simulink model "car_model_FIXED"  (R2022b)
settings: Solver=VariableStepAuto  StartTime=0.0  StopTime=60  RelTol=1e-3
values from neighbouring files (symbols this model uses):
  ABS_MAX_TORQUE = [25 25 25 25]    [workspace.mat]
  ABS_MAX_TRQ_CMD = 50    [workspace.mat]
  ABS_MIN_TORQUE = [0.01 0.01 0.01 0.01]    [workspace.mat]
  acc_IC = 0    [workspace.mat]
  ACCELERATION_MAX = 30    [workspace.mat]
  ActSuspDutyCycle = 1    [workspace.mat]
  Aeq_left = [0.305756190204 0.308857786592 0.311945941182 0.315020811431 0.318082554689 0.321131328186 0.324167289011 0.327190594103 0.330201400225 0.333199863958 0.336186141681 0.339160389558 ... (261 elements, 1x261)]    [workspace.mat]
  Aeq_right = [-0.961664782545 -0.959835898365 -0.957982924115 -0.956106413788 -0.954206913862 -0.952284963337 -0.950341093764 -0.948375829284 -0.946389686656 -0.944383175301 -0.942356797333 -0.940311047601 ... (261 elements, 1x261)]    [workspace.mat]
  alpha_error = 0.1    [workspace.mat]
  ang_acc_hystersesis = 0.1    [workspace.mat]
  ang_IC = 0    [workspace.mat]
  ang_vel_IC = 0    [workspace.mat]
  area_air = 0.15    [workspace.mat]
  axb = -5    [workspace.mat]
  battery_current_IC = 0    [workspace.mat]
  BATTERY_CURRENT_MAX = 140    [workspace.mat]
  BATTERY_CURRENT_MIN = 0    [workspace.mat]
  battery_FT_IC = 300    [workspace.mat]
  battery_T_IC = 300    [workspace.mat]
  BATTERY_TEMPERATURE_MAX = 60    [workspace.mat]
  BATTERY_TEMPERATURE_MIN = 0    [workspace.mat]
  battery_voltage_IC = 332    [workspace.mat]
  BATTERY_VOLTAGE_MAX = 340    [workspace.mat]
  BATTERY_VOLTAGE_MIN = 60    [workspace.mat]
  br = 0.01    [workspace.mat]
  brake_bias = [0.35 0.35 0.15 0.15]    [workspace.mat]
  Brake_Pressure_IC = 1    [workspace.mat]
  ccl_IC = 0    [workspace.mat]
  CENTER_STEER_ANGLE_MAX = 130    [workspace.mat]
  covarience_matrix_IC = [0.001 0 0 0 0 0 0 0 0 0 0 0 ... (784 elements, 28x28)]    [workspace.mat]
  CURRENT_BUFFER = 25    [workspace.mat]
  cy_sweep = [13568.4166816 14020.2069783 14456.754831 14879.7402576 15289.7264712 15687.2766846 16072.954111 16447.3219632 16810.9434544 17164.3817975 17508.2002054 17842.9618912 ... (101 elements, 1x101)]    [workspace.mat]
  dB = 0.001    [workspace.mat]
  dcl_IC = 140    [workspace.mat]
  DCL_MAX = 130    [workspace.mat]
  DCL_MIN = 0    [workspace.mat]
  deadband_angle = 12    [workspace.mat]
  dIndex = 50    [workspace.mat]
  driver_t = 0.015    [workspace.mat]
  dt_OFF = 4.5    [workspace.mat]
  dt_ON = 7.5    [workspace.mat]
  dTx = 0.01    [workspace.mat]
  dx = 0.1    [workspace.mat]
  dZ = 0.295    [workspace.mat]
  efficiency_grid = [0.759500051293 0.787587791453 0.809832189108 0.826747821898 0.837164543102 0.842744381136 0.842258400104 0.838611650621 0.82826195101 0.814029316176 0.795690627225 0.7759791486 ... (2782 elements, 26x107)]    [workspace.mat]
  F0z = [0 0]    [workspace.mat]
  forward_look_straight = 5    [workspace.mat]
  forward_look_turn = 15    [workspace.mat]
  Fz_IC = 539.55    [workspace.mat]
  Fz_sweep = [200 210 220 230 240 250 260 270 280 290 300 310 ... (101 elements, 1x101)]    [workspace.mat]
  g = 9.81    [workspace.mat]
  GAIN_ABS = 100    [workspace.mat]
  gearbox_efficiency = [0.8 0.8 0.8 0.8]    [workspace.mat]
  gps_counter_IC = 0    [workspace.mat]
  gps_hz = 0.01    [workspace.mat]
  gr = [8.74786324786 8.74786324786 8.74786324786 8.74786324786]    [workspace.mat]
  I = 0    [workspace.mat]
  I_Driver = 1    [workspace.mat]
  indicies = [3 3.5 4 0.5 1 1.5 2 2.5 3 3.5 4 0.5 ... (27 elements, 1x27)]    [workspace.mat]
  IYY = 0.3    [workspace.mat]
  kx_sweep = [8779.958 9178.302 9576.646 9974.99 10373.334 10771.678 11170.022 11568.366 11966.71 12365.054 12763.398 13161.742 ... (101 elements, 1x101)]    [workspace.mat]
  l = [0.772 0.772]    [workspace.mat]
  lambda_star = 0.15    [workspace.mat]
  low_V_SA = 0.001    [workspace.mat]
  lr = 35    [workspace.mat]
  m_all = 220    [workspace.mat]
  m_body = 180    [workspace.mat]
  m_unsprung = [6 6 14 14]    [workspace.mat]
  MAG_MAX = 200    [workspace.mat]
  Max_Brake_Pressure = 100000000    [workspace.mat]
  Max_Driver_Input = 1    [workspace.mat]
  MAX_DTHETA_DRIVER = 360    [workspace.mat]
  MAX_I_Driver = 1    [workspace.mat]
  MAX_STEERING_ADJUST = 15    [workspace.mat]
  max_yaw = [0.705271610162 0.928228152446 1.12280857731 1.14131008363 1.08727026041 1.01377803859 0.938114723816 0.8718206875 0.815009168116 0.767481919497 0.727119764215 0.694403589394 ... (15 elements, 1x15)]    [workspace.mat]
  Min_Brake_Pressure = 1    [workspace.mat]
  Min_Driver_Input = 0    [workspace.mat]
  min_velocity_regen = 1.4    [workspace.mat]
  motor_current_IC = 0    [workspace.mat]
  MOTOR_CURRENT_MAX = 70    [workspace.mat]
  MOTOR_CURRENT_MIN = 0    [workspace.mat]
  MOTOR_ENABLE = [0 0 1 1]    [workspace.mat]
  motor_FT_IC = 300    [workspace.mat]
  motor_T_IC = 300    [workspace.mat]
  MOTOR_TEMPERATURE_MAX = 100    [workspace.mat]
  MOTOR_TEMPERATURE_MIN = 0    [workspace.mat]
  motor_voltage_IC = 332    [workspace.mat]
  MOTOR_VOLTAGE_MAX = 340    [workspace.mat]
  MOTOR_VOLTAGE_MIN = 90    [workspace.mat]
  motorControllerCurve = [25  260; 50  130; 75  0]    [workspace.mat]
  motorTempCurve = [140 138.6 134.4 127.4 117.6 105 89.6 71.4 50.4 26.6 0]    [workspace.mat]
  motorTempX = [75 77 79 81 83 85 87 89 91 93 95]    [workspace.mat]
  mu_star = 0.5    [workspace.mat]
  mx_sweep = [3.38348 3.3655067 3.3477908 3.3303323 3.3131312 3.2961875 3.2795012 3.2630723 3.2469008 3.2309867 3.21533 3.1999307 ... (101 elements, 1x101)]    [workspace.mat]
  my_sweep = [3.036232 3.015241699 2.994987032 2.975452753 2.956623616 2.938484375 2.921019784 2.904214597 2.888053568 2.872521451 2.857603 2.843282969 ... (101 elements, 1x101)]    [workspace.mat]
  noise_state = [1e-06 1e-06 1e-06 1e-06 0.005 0.005 0.005 1e-06 1e-06 1e-06 1e-06 1e-06 ... (28 elements, 28x1)]    [workspace.mat]
  omega_IC = 0    [workspace.mat]
  OMEGA_MAX = 150    [workspace.mat]
  OMEGA_MIN = 0    [workspace.mat]
  ORIENTATION_MAX = 360    [workspace.mat]
  P = 2    [workspace.mat]
  P_Driver = 0.7    [workspace.mat]
  P_High_Speed = 0.1    [workspace.mat]
  P_Steering_Adjust = 2    [workspace.mat]
  P_Straight_Adjust = 5    [workspace.mat]
  pos_IC = 0    [workspace.mat]
  POS_MAX = 300    [workspace.mat]
  q_thresh = 0.3    [workspace.mat]
  RE = 0.223    [workspace.mat]
  rho = 1.225    [workspace.mat]
  s = [0.649 0.621]    [workspace.mat]
  selected_maxvm = [49.86390724 16.21289794 8.219813569 8.05215527 7.103352929 8.35634983 13.87515039 8.72402841 22.75224945 36.67909339 19.32001297 25.09036962 ... (63 elements, 21x3)]    [workspace.mat]
  selected_sweep = [3 3 3 3 3 3 3 3 3 3 3 3 ... (1288 elements, 644x2)]    [workspace.mat]
  selected_track = [inf inf inf inf inf inf inf inf inf inf inf inf ... (37971 elements, 4219x9)]    [workspace.mat]
  shock_length_IC = 0.1    [workspace.mat]
  SHOCK_LENGTH_MAX = 0.25    [workspace.mat]
  SHOCK_LENGTH_MIN = 0    [workspace.mat]
  state_IC = [1 0 0 0 0 0 0 0 0 0 0 0 ... (28 elements, 28x1)]    [workspace.mat]
  steering_sweep = [0 5 10 15 20 25 30 35 40 45 50 55 ... (27 elements, 1x27)]    [workspace.mat]
  steering_Up_Grid = [0.551231966244 8.36038106007 16.1333806643 23.9559539118 31.8240691982 39.7561724339 47.7157531433 55.7845698794 64.1341708168 73.0798046026 82.7903081349 93.1297322155 ... (615 elements, 41x15)]    [workspace.mat]
  ... (+25 more)
undefined symbols (not defined in the file or in its folder): ax, ay, az, covA, covG, covM, covP, covV, DiscIntNeverNeededParam, fusion_t, fusion_t_sim, gps_ratio, IMU_accel, IMU_gyro, imu_hz, IMU_mag, location_lla_IC, p, phi, psi, q, r, sus, theta, trn, veh, VEH, whl, X, Xdot, Y, Ydot, Z, Zdot
libraries: fl_lib x82, nesl_utility x32, vehdynlibtire x10, vehdynlibsuspension x8, simulink x5, autolibutils x5, sharedtransform x5, sdl_lib x4, EngineCoolingComponents_lib x4, slpidlib x3, SimscapeFluids_lib x3, shared6dof x2
(part 4 of 14)

== system car_model_FIXED/Vehicle Model/Suspension ==
  Steering : Inport
  Wheel : Inport  Port=2
  Vehicle : Inport  Port=3
  Double Wishbone Suspension : Subsystem  VariantControl=1
      mask Display: image('suspdw.png');
  Independent Mapped Front Suspension Mapped Solid Axle Rear Suspension : Subsystem  VariantControl=2
      mask Display: image([imread('suspindmap.png');imread('suspsamap.png')]);
  Kinematics and Compliance Independent Suspension : Subsystem  VariantControl=6
      mask Display: image('suspkandc.png');
  MacPherson Front Suspension Solid Axle Rear Suspension : Subsystem  VariantControl=3
      mask Display: image([imread('suspmacp.png');imread('suspsacoil.png')]);
  MacPherson Suspension : Subsystem  VariantControl=4
      mask Display: image('suspmacp.png');
  Mapped Suspension : Subsystem  VariantControl=5
      mask Display: image('suspindmap.png');
  Suspension : Outport  VectorParamsAs1DForOutWhenUnconnected=off
  Suspension1 : Outport  Port=2  VectorParamsAs1DForOutWhenUnconnected=off
  Veh : Outport  Port=3  VectorParamsAs1DForOutWhenUnconnected=off

== system car_model_FIXED/Vehicle Model/Vehicle ==
  Suspension : Inport
  6DOF : Subsystem  VariantControl=1
  Constant : Constant  Value=[0 0 0]
  VehFdbk : Outport  VectorParamsAs1DForOutWhenUnconnected=off
  wires:
  6DOF/1(VehFdbk) -> VehFdbk/1  "VehFdbk"
  Constant/1 -> 6DOF/2(Wind)
  Suspension/1 -> 6DOF/1(Suspension)

== system car_model_FIXED/Vehicle Model/Wheels and Tires ==
  Brake Press : Inport  Unit=Pa
  PwrTrn : Inport  Port=2
  Sus : Inport  Port=3
  Veh : Inport  Port=4
  Bus Selector : BusSelector  OutputSignals=axle_torque
  Bus Selector1 : BusSelector  OutputSignals=Whl.Ang,Whl.F,Whl.AngVel,Whl.xdot,Whl.ydot
  Bus Selector2 : BusSelector  OutputSignals=BdyFrm.Cg.Vel.xdot,BdyFrm.Cg.Vel.ydot  OutputAsBus=on
  Constant1 : Constant  Value=[1 1 1 1].*0.00182
  Constant3 : Constant  Value=[1 1 1 1]
  Cont LPF : autolibutils/Cont LPF  wc=100*2*pi  AbsoluteTolerance=auto  aMode=2
  Cont LPF1 : autolibutils/Cont LPF  wc=100*2*pi  AbsoluteTolerance=auto  aMode=2
  Matrix Concatenate : Concatenate  NumInputs=3  Mode=Multidimensional array
  Reshape{1..4} (4 alike) : Reshape
  Saturation : Saturate  UpperLimit=inf  LowerLimit=-10*9.81*2000  ZeroCross=off
  Selector : Selector  NumberOfDimensions=2  InputPortWidth=3  IndexOptions=Index vector (dialog),Select all  Indices=[3],1  OutputSizes=1,1
  Selector1 : Selector  NumberOfDimensions=2  InputPortWidth=1  IndexOptions=Index vector (dialog),Select all  Indices=[3],1  OutputSizes=1,1
  Selector2 : Selector  NumberOfDimensions=2  InputPortWidth=3  IndexOptions=Index vector (dialog),Select all  Indices=3,1  OutputSizes=1,1
  Selector3 : Selector  NumberOfDimensions=2  InputPortWidth=3  IndexOptions=Index vector (dialog),Select all  Indices=1,1  OutputSizes=1,1
  Sqrt : Sqrt
  Square : Math  Operator=square
  Sum : Sum  Inputs=+
  Terminator{,1..2,4..5} (5 alike) : Terminator
  VDBS : Subsystem  VariantControl=0
  Vehicle : Outport  VectorParamsAs1DForOutWhenUnconnected=off
  Suspension : Outport  Port=2  VectorParamsAs1DForOutWhenUnconnected=off
  Wheels : Outport  Port=3  VectorParamsAs1DForOutWhenUnconnected=off
  Power Train : Outport  Port=4  VectorParamsAs1DForOutWhenUnconnected=off
  Wheels2Susp : Outport  Port=5  VectorParamsAs1DForOutWhenUnconnected=off
  Vg : Outport  Port=6  VectorParamsAs1DForOutWhenUnconnected=off
  wires:
  Bus Selector1/2 -> Selector/1  "<F>"
  VDBS/3(FrntAxlF) -> Terminator/1
  VDBS/4(RearAxlF) -> Terminator1/1
  VDBS/6(Mz) -> Terminator4/1
  Selector1/1 -> Reshape1/1
  Matrix Concatenate/1 -> VDBS/7(VehVel)
  PwrTrn/1 -> Power Train/1, Bus Selector/1
  Reshape4/1 -> VDBS/1(WhlAng)  "WhlAng"
  Reshape3/1 -> VDBS/2(WhlCmb)  "WhlCmb"
  Selector/1 -> Reshape2/1
  Saturation/1 -> VDBS/5(Fz)
  Constant1/1 -> VDBS/8(Ground Level)
  VDBS/8(SuspWhlVz) -> Matrix Concatenate/3  "zdot"
  Bus Selector1/1 -> Cont LPF1/1  "<Ang>"
  Selector3/1 -> Reshape3/1  "Camber Angles"
  Sus/1 -> Suspension/1, Bus Selector1/1
  Bus Selector1/4 -> Matrix Concatenate/1  "<xdot>"
  Bus Selector1/5 -> Matrix Concatenate/2  "<ydot>"
  VDBS/7(SuspWhlPz) -> Terminator5/1  "z"
  Reshape2/1 -> Cont LPF/1
  Bus Selector1/3 -> Selector1/1  "<AngVel>"
  Reshape1/1 -> VDBS/6(r)
  Brake Press/1 -> VDBS/4(BrkPed)
  Constant3/1 -> VDBS/9(Friction)
  Cont LPF/1 -> Saturation/1
  Cont LPF1/1 -> Selector3/1, Selector2/1
  Selector2/1 -> Reshape4/1  "Wheel Angles"
  Veh/1 -> Vehicle/1, Bus Selector2/1, VDBS/10(Veh)  "Veh"
  VDBS/2(Wheels2Susp) -> Wheels2Susp/1  "Wheels"
  VDBS/1(Wheels) -> Wheels/1
  Bus Selector/1 -> VDBS/3(AxleTrq)  "<axle_torque>"
  VDBS/5(Omega) -> Terminator2/1
  Bus Selector2/1 -> Square/1
  Square/1 -> Sum/1
  Sum/1 -> Sqrt/1
  Sqrt/1 -> Vg/1

== system car_model_FIXED/Control Systems/TVS/Optimization ==
  note: reduce this limit?
  driver_input : Inport  OutDataTypeStr=double
  obj_gain : Inport  Port=2
  b : Inport  Port=3  OutDataTypeStr=double
  ub : Inport  Port=4  OutDataTypeStr=double
  lb : Inport  Port=5  OutDataTypeStr=double
  Aeq : Inport  Port=6  OutDataTypeStr=double
  beq : Inport  Port=7  OutDataTypeStr=double
  A Dot : DotProduct  OutDataTypeStr=double
  Aeq Dot : DotProduct  OutDataTypeStr=double
  C Caller : CCaller  FunctionName=bigM_func  PortSpecificationStruct="%)30     .    N\"X   8    (     @         %    \"    !P    !     0         %  0 \"0    $    _    07)G3F%M90  4&]R=$YA;64 4V-O<&4     26YD97@     5'EP90      4VEZ90      27-';&]B86P   X    P    !@    @    $          4    (     0    ,    !         !   P!O=70 #@   #     &    \"     0         !0    @    !     P    $         $  # &]U=  .    .     8    (    !          %    \"     $    &     0         0  ...(+15750 chars)"
  Constant : Constant  Value=TVS_ENABLE
  Constant1 : Constant  Value=[1 1 1 1]
  Demux{,1..4} (5 alike) : Demux
  Switch : Switch  Criteria=u2 > Threshold  SaturateOnIntegerOverflow=off  InputSameDT=off
  Tx_RAW_demux : Mux
  Tx_choose : Switch  Criteria=u2 > Threshold  Threshold=2  OutDataTypeStr=double  SaturateOnIntegerOverflow=off  InputSameDT=off
  Tx_deadband : DeadZone  LowerValue=-10*dTx  UpperValue=10*dTx  SaturateOnIntegerOverflow=off
  Tx_equal_gain : Gain  Gain=ABS_MAX_TORQUE.*MOTOR_ENABLE  OutDataTypeStr=double
  Tx_equal_offset : Bias  Bias=ABS_MAX_TORQUE  SaturateOnIntegerOverflow=off
  Tx_initial : Constant  Value=Tx_I  OutDataTypeStr=double
  Tx_rate_limit : RateLimiter  RisingSlewLimit=Torque_Up_Rate_Limit  FallingSlewLimit=-Torque_Down_Rate_Limit  SampleTimeMode=inherited
  Tx_reverse_offset : Bias  Bias=-ABS_MAX_TORQUE  SaturateOnIntegerOverflow=off
  b Add : Sum  OutDataTypeStr=double
  beq Add : Sum  OutDataTypeStr=double
  lb_offset : Bias  Bias=ABS_MAX_TORQUE  SaturateOnIntegerOverflow=off
  optimization_offset_A : Constant  Value=ABS_MAX_TORQUE  OutDataTypeStr=double
  optimization_offset_Aeq : Constant  Value=ABS_MAX_TORQUE  OutDataTypeStr=double
  ub_offset : Bias  Bias=ABS_MAX_TORQUE  SaturateOnIntegerOverflow=off
  yaw_error_limit : Constant  Value=yaw_error_limit  OutDataTypeStr=double
  Tx : Outport
  exitflag : Outport  Port=2
  wires:
  C Caller/1 -> Tx_choose/2, exitflag/1  "exitflag"
  lb/1 -> lb_offset/1  "lb"
  ub/1 -> ub_offset/1  "ub"
  C Caller/2 -> Tx_RAW_demux/1  "TFL"
  C Caller/5 -> Tx_RAW_demux/4  "TRR"
  C Caller/4 -> Tx_RAW_demux/3  "TRL"
  C Caller/3 -> Tx_RAW_demux/2  "TFR"
  Demux/1 -> C Caller/1  "obj_FL"
  Demux/2 -> C Caller/2  "obj_FR"
  Demux/3 -> C Caller/3  "obj_RL"
  Demux/4 -> C Caller/4  "obj_RR"
  Tx_initial/1 -> C Caller/23, C Caller/24, C Caller/26, C Caller/25  "Tx_initial"
  Demux1/1 -> C Caller/19  "ub_FL"
  Demux1/2 -> C Caller/20  "ub_FR"
  Demux1/3 -> C Caller/21  "ub_RL"
  Demux1/4 -> C Caller/22  "ub_RR"
  Demux2/1 -> C Caller/15  "lb_FL"
  Demux2/2 -> C Caller/16  "lb_FR"
  Demux2/3 -> C Caller/17  "lb_RL"
  Demux2/4 -> C Caller/18  "lb_RR"
  Demux3/3 -> C Caller/13  "Aeq_RL"
  Demux3/2 -> C Caller/12  "Aeq_FR"
  Demux3/1 -> C Caller/11  "Aeq_FL"
  Demux3/4 -> C Caller/14  "Aeq_RR"
  Demux4/1 -> C Caller/6  "A_FL"
  Demux4/2 -> C Caller/7  "A_FR"
  Demux4/3 -> C Caller/8  "A_RL"
  Demux4/4 -> C Caller/9  "A_RR"
  ub_offset/1 -> Demux1/1  "ub_b"
  optimization_offset_Aeq/1 -> Aeq Dot/1  "offset"
  optimization_offset_A/1 -> A Dot/1  "offset"
  beq/1 -> beq Add/1  "beq"
  Aeq Dot/1 -> beq Add/2  "Aeq_b"
  b/1 -> b Add/1  "b"
  A Dot/1 -> b Add/2
  yaw_error_limit/1 -> C Caller/27  "yaw_error_limit"
  Tx_RAW_demux/1 -> Tx_choose/1  "Tx_RAW_TV"
  Constant1/1 -> Demux4/1, A Dot/2  "A"
  b Add/1 -> C Caller/5  "b_b"
  obj_gain/1 -> Demux/1  "obj_gain"
  lb_offset/1 -> Demux2/1  "lb_b"
  Aeq/1 -> Demux3/1, Aeq Dot/2  "Aeq"
  beq Add/1 -> C Caller/10  "beq_b"
  Tx_rate_limit/1 -> Tx/1  "Tx"
  Tx_reverse_offset/1 -> Tx_deadband/1
  driver_input/1 -> Tx_equal_gain/1
  Tx_deadband/1 -> Tx_rate_limit/1
  Tx_choose/1 -> Switch/1
  Tx_equal_gain/1 -> Tx_equal_offset/1  "Tx_equal"
  Tx_equal_offset/1 -> Switch/3, Tx_choose/3
  Switch/1 -> Tx_reverse_offset/1
  Constant/1 -> Switch/2

== system car_model_FIXED/Control Systems/TVS/Power Controller ==
  note: Tune the distance before PL is enabled
  note: Create a better map wherein you have T,V,I,w
  note: Tune the endpoints
  vel : Inport  OutDataTypeStr=double
  battery_voltage : Inport  Port=2
  pack_current : Inport  Port=3
  dcl : Inport  Port=4  OutDataTypeStr=double  LockScale=on
  ccl : Inport  Port=5  OutDataTypeStr=double  LockScale=on
  driver_input : Inport  Port=6  OutDataTypeStr=double  LockScale=on
  motor_temp : Inport  Port=7
  mc_temp : Inport  Port=8
  omega : Inport  Port=9
  Abs Max Torque CMD (Nm) : Constant  Value=ABS_MAX_TRQ_CMD
  Constant2 : Constant  Value=[0 0 0 0]  OutDataTypeStr=double
  Constant3 : Constant  Value=ABS_MAX_TORQUE
  Current to Torque : Gain  Gain=ABS_MAX_TRQ_CMD/BATTERY_CURRENT_MAX
  Gain4 : Gain  Gain=-MOTOR_ENABLE  ParamDataTypeStr=double  OutDataTypeStr=Inherit: Inherit via back propagation
  Gain8 : Gain  Gain=MOTOR_ENABLE  ParamDataTypeStr=double  OutDataTypeStr=Inherit: Inherit via back propagation
  Max : MinMax  Function=max
  Max Torque : Saturate  UpperLimit=ABS_MAX_TORQUE  LowerLimit=dTx  OutDataTypeStr=Inherit: Inherit via back propagation
  Max Torque Command Selector : Switch  Criteria=u2 > Threshold  Threshold=CURRENT_BUFFER  SaturateOnIntegerOverflow=off  InputSameDT=off
  Max1 : MinMax  Function=max
  Min Throttle Command (Nm) : Constant  Value=dTx*10
  Min Torque : Saturate  UpperLimit=ABS_MIN_TORQUE  LowerLimit=0  OutDataTypeStr=Inherit: Inherit via back propagation
  Minimum : MinMax  Inputs=3
  Selector : Selector  InputPortWidth=4  IndexOptions=Index vector (dialog)  Indices=4  OutputSizes=1
  Subtract : Sum  Inputs=+-
  Switch1 : Switch  Threshold=min_velocity_regen  OutDataTypeStr=Inherit: Inherit via back propagation  SaturateOnIntegerOverflow=off  InputSameDT=off
  Temperature to Motor Controller Current Limit Map : Lookup_n-D  NumberOfTableDimensions=1  BreakpointsForDimension1=motorControllerCurve(:,1)  IndexSearchMethod=Evenly spaced points  Table=motorControllerCurve(:,2)  ExtrapMethod=Clip  UseLastTableValue=on  InternalRulePriority=Speed  RndMeth=Simplest
  Temperature to Motor Current Limit Map : Lookup_n-D  NumberOfTableDimensions=1  BreakpointsForDimension1=motorTempX  IndexSearchMethod=Evenly spaced points  Table=motorTempCurve  ExtrapMethod=Clip  UseLastTableValue=on  InternalRulePriority=Speed  RndMeth=Simplest
  Terminator : Terminator
  Terminator1 : Terminator
  Terminator2 : Terminator
  "Throttle Map " : Lookup_n-D  NumberOfTableDimensions=1  BreakpointsForDimension1=throttleX  IndexSearchMethod=Evenly spaced points  Table=throttleCurve  ExtrapMethod=Clip  InternalRulePriority=Speed  RndMeth=Simplest
  Throttle Saturation : simulink/Discontinuities/Saturation Dynamic  OutMin=[0]  OutMax=[]  OutDataTypeStr=Inherit: Same as second input  OutDataType=fixdt(1, 16)  OutScaling=2^-10  DoSatur=off
  Throttle to Torque : Gain  Gain=ABS_MAX_TRQ_CMD
  b : Outport  OutDataTypeStr=double  LockScale=on
  Max b : Outport  Port=2  OutDataTypeStr=double  LockScale=on
  ub : Outport  Port=3  OutDataTypeStr=double  LockScale=on
  lb : Outport  Port=4  OutDataTypeStr=double  LockScale=on
  wires:
  Max1/1 -> Temperature to Motor Controller Current Limit Map/1
  Temperature to Motor Current Limit Map/1 -> Minimum/2  "Total Motor Current Limit (A)"
  battery_voltage/1 -> Terminator1/1
  Min Throttle Command (Nm)/1 -> Throttle Saturation/3
  Gain8/1 -> Max Torque/1
  Constant3/1 -> Gain4/1, Gain8/1
  Throttle Saturation/1 -> b/1  "Limited Torque CMD (Nm)"
  Max/1 -> Temperature to Motor Current Limit Map/1
  Gain4/1 -> Min Torque/1
  Constant2/1 -> Switch1/3  "Abs Min Torque CMD"
  Selector/1 -> Switch1/2  "Planer Vcog (m/s)"
  motor_temp/1 -> Max/1  "[FL FR RL RR] Motor Temperature (degC)"
  ccl/1 -> Terminator/1
  driver_input/1 -> "Throttle Map "/1  "RAW Throttle"
  Max Torque/1 -> ub/1  "Max Individual Motor Torque (Nm)"
  "Throttle Map "/1 -> Throttle to Torque/1  "Mapped Throttle"
  Throttle to Torque/1 -> Throttle Saturation/2  "RAW Torque CMD (Nm)"
  mc_temp/1 -> Max1/1  "[FL FR RL RR] Motor Controller Temperature (degC)"
  dcl/1 -> Minimum/1  "Discharge Current Limit (A)"
  vel/1 -> Selector/1  "[Vx Vy Vcog]"
  Temperature to Motor Controller Current Limit Map/1 -> Minimum/3  "Total Motor Controller Current Limit (A)"
  Min Torque/1 -> Switch1/1
  Switch1/1 -> lb/1  "Min Individual Motor Torque (Nm)"
  Subtract/1 -> Max Torque Command Selector/2  "Distance to DCL (A)"
  Abs Max Torque CMD (Nm)/1 -> Max Torque Command Selector/1
  Current to Torque/1 -> Max Torque Command Selector/3  "Temperature Dependent Max Torque CMD (Nm)"
  pack_current/1 -> Subtract/2  "pack_current (A)"
  Minimum/1 -> Current to Torque/1, Subtract/1  "Max Allowed Pack Current (A)"
  Max Torque Command Selector/1 -> Max b/1, Throttle Saturation/1  "Max Allowed Torque CMD (Nm)"
  omega/1 -> Terminator2/1

== system car_model_FIXED/Control Systems/TVS/Traction Controller ==
  Fz : Inport  OutDataTypeStr=double  LockScale=on
  vel : Inport  Port=2  OutDataTypeStr=double  LockScale=on
  ang_vel : Inport  Port=3  OutDataTypeStr=double  LockScale=on
  CCSA : Inport  Port=4
  omega : Inport  Port=5
  1-D Lookup Table : Lookup_n-D  NumberOfTableDimensions=1  BreakpointsForDimension1=Fz_sweep  Table=cy_sweep  InternalRulePriority=Speed  RndMeth=Simplest
  1-D Lookup Table1 : Lookup_n-D  NumberOfTableDimensions=1  BreakpointsForDimension1=Fz_sweep  Table=my_sweep  InternalRulePriority=Speed  RndMeth=Simplest
  1-D Lookup Table2 : Lookup_n-D  NumberOfTableDimensions=1  BreakpointsForDimension1=Fz_sweep  Table=kx_sweep  InternalRulePriority=Speed  RndMeth=Simplest
  1-D Lookup Table3 : Lookup_n-D  NumberOfTableDimensions=1  BreakpointsForDimension1=Fz_sweep  Table=mx_sweep  InternalRulePriority=Speed  RndMeth=Simplest
  Compute SA : Subsystem
  Compute SL : Subsystem
  Compute SL Fake : Subsystem
  Constant : Constant
  Constant1 : Constant  Value=[1 1 1 1].*low_V_SA
  Constant2 : Constant  Value=TRACTION_ENABLE
  Divide : Product  Inputs=**//
  Divide1 : Product  Inputs=**//
  Gain : Gain  Gain=gr./RE
  Selector : Selector  InputPortWidth=4  IndexOptions=Index vector (dialog)  Indices=4  OutputSizes=1
  Selector1 : Selector  InputPortWidth=4  IndexOptions=Index vector (dialog)  Indices=4  OutputSizes=1
  Sqrt : Sqrt
  Square : Math  Operator=square
  Square1 : Math  Operator=square
  Steering Model : Subsystem
  Sum : Sum  Inputs=|++
  Switch : Switch  Criteria=u2 > Threshold  Threshold=Vth  SaturateOnIntegerOverflow=off  InputSameDT=off
  Switch1 : Switch  Criteria=u2 > Threshold  Threshold=Vth  SaturateOnIntegerOverflow=off  InputSameDT=off
  Switch2 : Switch  Criteria=u2 > Threshold  SaturateOnIntegerOverflow=off  InputSameDT=off
  obj_gain : Outport
  wires:
  Gain/1 -> obj_gain/1  "obj_gain"
  Constant/1 -> Gain/1, Switch2/3
  Sum/1 -> Sqrt/1
  Divide/1 -> Square/1  "a_bar"
  1-D Lookup Table/1 -> Divide/2
  1-D Lookup Table1/1 -> Divide/3
  Fz/1 -> 1-D Lookup Table1/1, Divide/4, 1-D Lookup Table2/1, 1-D Lookup Table3/1, Divide1/4, 1-D Lookup Table/1
  Divide1/1 -> Square1/1  "s_bar"
  1-D Lookup Table2/1 -> Divide1/2
  1-D Lookup Table3/1 -> Divide1/3
  Switch/1 -> Divide1/1
  Switch1/1 -> Divide/1
  Compute SL Fake/1(SL_fake) -> Switch/3
  Compute SL/1(Out1) -> Switch/1
  Compute SA/1(Out1) -> Switch1/1, Compute SL/1(In1)
  vel/1 -> Compute SL/3(Vg), Selector/1, Compute SL Fake/2(Vg), Selector1/1, Compute SA/3(Vg)
  ang_vel/1 -> Compute SA/2(ang_vel)
  omega/1 -> Compute SL Fake/1(omega), Compute SL/2(omega)
  Steering Model/1(steering) -> Compute SA/1(steering)
  Constant1/1 -> Switch1/3
  Sqrt/1 -> Switch2/1
  Constant2/1 -> Switch2/2
  Selector/1 -> Switch/2
  Selector1/1 -> Switch1/2
  Square/1 -> Sum/1
  Square1/1 -> Sum/2
  CCSA/1 -> Steering Model/1(steering_angle)

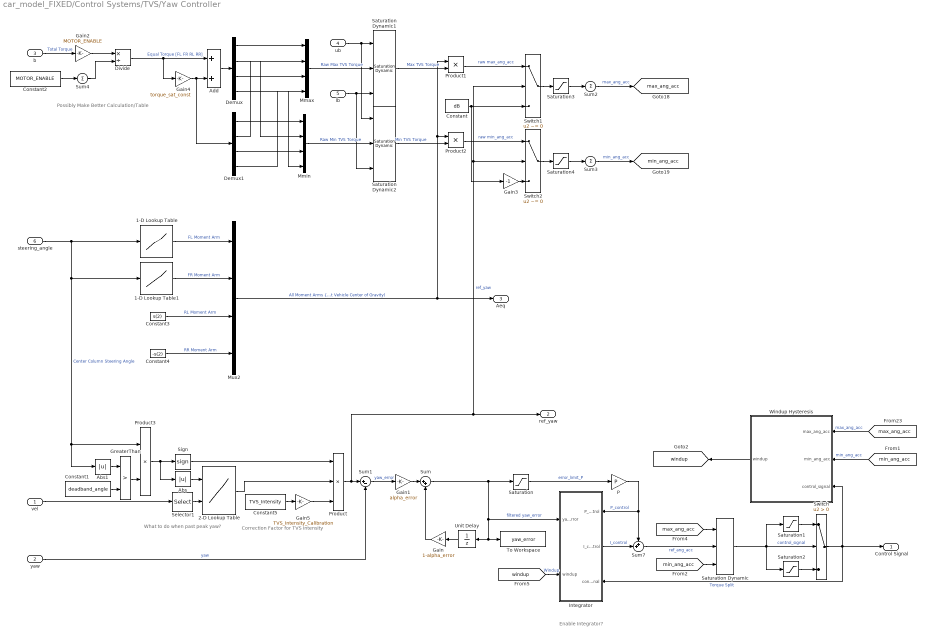
== system car_model_FIXED/Control Systems/TVS/Yaw Controller ==
  note: Correction Factor for TVS Intensity
  note: Enable Integrator?
  note: What to do when past peak yaw?
  note: Possibly Make Better Calculation/Table
  vel : Inport
  yaw : Inport  Port=2  OutDataTypeStr=double  LockScale=on
  b : Inport  Port=3
  ub : Inport  Port=4
  lb : Inport  Port=5
  steering_angle : Inport  Port=6
  1-D Lookup Table : Lookup_n-D  NumberOfTableDimensions=1  BreakpointsForDimension1=theta_sweep  Table=Aeq_left  ExtrapMethod=Clip  InternalRulePriority=Speed  RndMeth=Simplest
  1-D Lookup Table1 : Lookup_n-D  NumberOfTableDimensions=1  BreakpointsForDimension1=theta_sweep  Table=Aeq_right  ExtrapMethod=Clip  InternalRulePriority=Speed  RndMeth=Simplest
  2-D Lookup Table : Lookup_n-D  BreakpointsForDimension1=steering_sweep  BreakpointsForDimension2=velocity_sweep  Table=yaw_rate  ExtrapMethod=Clip  InternalRulePriority=Speed  RndMeth=Simplest
      settings: InputPortMap=u0,u1
  Abs : Abs  SaturateOnIntegerOverflow=off
  Abs1 : Abs  SaturateOnIntegerOverflow=off
  Add : Sum
  Constant : Constant  Value=dB  OutDataTypeStr=Inherit: Inherit via back propagation
  Constant1 : Constant  Value=deadband_angle
  Constant2 : Constant  Value=MOTOR_ENABLE
  Constant3 : Constant  Value=s(2)  OutDataTypeStr=Inherit: Inherit via back propagation
  Constant4 : Constant  Value=-s(2)  OutDataTypeStr=Inherit: Inherit via back propagation
  Constant5 : Constant  Value=TVS_Intensity
  Demux : Demux
  Demux1 : Demux
  Divide : Product  Inputs=*/
  Gain : Gain  Gain=1-alpha_error
  Gain1 : Gain  Gain=alpha_error
  Gain2 : Gain  Gain=MOTOR_ENABLE
  Gain3 : Gain  Gain=-1
  Gain4 : Gain  Gain=torque_sat_const
  Gain5 : Gain  Gain=TVS_Intensity_Calibration
  GreaterThan : RelationalOperator  Operator=>  OutDataTypeStr=boolean  RndMeth=Simplest  InputSameDT=off
  Integrator : Subsystem
      settings: PortSchema="{\"entries\":[{\"content\":{\"sides\":[{\"content\":{\"connectorIds\":[\"In1\",\"In2\"]},\"type\":\"ConnectorPlacement.EquallySpacedRectSide\",\"uuid\":\"8eceed30-5463-482b-9ad9-1d0859eec1e0\"},{\"content\":{\"connectorIds\":[\"In3\",\"Out1\",\"In4\"],\"side\":\"RIGHT\"},\"type\":\"ConnectorPlacement.EquallySpacedRectSide\",\"uuid\":\"ca18b8b2-b2b4-4da4-8362-ca68ae703b33\"},{\"content\":{\"connectorIds\":[],\"side\":\"TOP\"},\"type\":\"ConnectorPlacement.EquallySpacedRectSide\",\"uuid\":\"14e81d29-e47e-408e-961b-b14eadc3d40e\"}]},\"type\":\"ConnectorPlacement.EquallySpacedConnector\",\"uuid\":\"147d3fcd-d0df-4d8b-910b-d1c7e2c77e1f\"}],\"packageUris\":[\"http://schema.mathworks.com/mf0/Connector/R2020b\"],\"version\":\"1.0\"}"
  Mmax : Mux
  Mmin : Mux
  Mux2 : Mux
  P : Gain  Gain=P  ParamDataTypeStr=double  OutDataTypeStr=double
  Product : Product  Inputs=3  OutDataTypeStr=Inherit: Inherit via back propagation
  Product1 : Product
  Product2 : Product
  Product3 : Product
  Saturation : Saturate  UpperLimit=YAW_MAX  LowerLimit=-YAW_MAX
  Saturation Dynamic : simulink/Discontinuities/Saturation Dynamic  OutMin=[]  OutMax=[]  OutDataTypeStr=Inherit: Same as second input  OutDataType=fixdt(1, 16)  OutScaling=2^-10  DoSatur=off
  Saturation Dynamic1 : simulink/Discontinuities/Saturation Dynamic  OutMin=[]  OutMax=[]  OutDataTypeStr=Inherit: Same as second input  OutDataType=fixdt(1, 16)  OutScaling=2^-10  DoSatur=off
  Saturation Dynamic2 : simulink/Discontinuities/Saturation Dynamic  OutMin=[]  OutMax=[]  OutDataTypeStr=Inherit: Same as second input  OutDataType=fixdt(1, 16)  OutScaling=2^-10  DoSatur=off
  Saturation1 : Saturate  UpperLimit=inf  LowerLimit=dB
  Saturation2 : Saturate  UpperLimit=-dB  LowerLimit=-inf
  Saturation3 : Saturate  UpperLimit=inf  LowerLimit=dB
  Saturation4 : Saturate  UpperLimit=-dB  LowerLimit=-inf
  Selector1 : Selector  InputPortWidth=4  IndexOptions=Index vector (dialog)  Indices=4  OutputSizes=1
  Sign : Signum
  Sum : Sum  Inputs=|++
  Sum1 : Sum  Inputs=|+-  OutDataTypeStr=Inherit: Inherit via back propagation
  Sum2 : Sum  Inputs=+
  Sum3 : Sum  Inputs=+
  Sum4 : Sum  Inputs=+
  Sum7 : Sum  Inputs=++|  OutDataTypeStr=double  SaturateOnIntegerOverflow=on
  Switch : Switch  Criteria=u2 > Threshold  SaturateOnIntegerOverflow=off  InputSameDT=off
  Switch1 : Switch  Criteria=u2 ~= 0  OutDataTypeStr=Inherit: Inherit via back propagation  SaturateOnIntegerOverflow=off  InputSameDT=off
  Switch2 : Switch  Criteria=u2 ~= 0  OutDataTypeStr=Inherit: Inherit via back propagation  SaturateOnIntegerOverflow=off  InputSameDT=off
  To Workspace : ToWorkspace  VariableName=yaw_error  SaveFormat=Timeseries  SampleTime=-1
  Unit Delay : UnitDelay  SampleTime=-1  HasFrameUpgradeWarning=on
  Windup Hysteresis : Subsystem
  Control Signal : Outport  OutDataTypeStr=double  PortDimensions=1  LockScale=on
  ref_yaw : Outport  Port=2
  Aeq : Outport  Port=3  OutDataTypeStr=double  LockScale=on
  tag scope: max_ang_acc=global, min_ang_acc=global, windup=global
  wires:
  P/1 -> Sum7/1, Integrator/3(P_control)  "P_control"
  yaw/1 -> Sum1/2  "yaw"
  Integrator/1(I_control) -> Sum7/2  "I_control"
  Sum7/1 -> Saturation Dynamic/2  "ref_ang_acc"
  Saturation Dynamic/1 -> Saturation2/1, Saturation1/1, Switch/2  "control_signal"
  Sum2/1 -> [max_ang_acc]  "max_ang_acc"
  Sum3/1 -> [min_ang_acc]  "min_ang_acc"
  Saturation/1 -> P/1  "error_limit_P"
  Windup Hysteresis/1(windup) -> [windup]
  Sum/1 -> Saturation/1, Unit Delay/1, To Workspace/1, Integrator/1(yaw_error)  "filtered yaw_error"
  [windup] -> Integrator/2(windup)  "Windup"
  Unit Delay/1 -> Gain/1
  Gain/1 -> Sum/2
  Gain1/1 -> Sum/1
  Sum1/1 -> Gain1/1  "yaw_error"
  Switch/1 -> Windup Hysteresis/3(control_signal), Control Signal/1, Integrator/4(control_signal)  "Torque Split"
  Saturation1/1 -> Switch/1
  Saturation2/1 -> Switch/3
  Saturation4/1 -> Sum3/1
  Gain3/1 -> Switch2/3
  Demux1/4 -> Mmax/4
  Constant4/1 -> Mux2/4  "RR Moment Arm"
  Switch2/1 -> Saturation4/1
  b/1 -> Gain2/1  "Total Torque"
  Constant3/1 -> Mux2/3  "RL Moment Arm"
  1-D Lookup Table/1 -> Mux2/1  "FL Moment Arm"
  Demux/3 -> Mmax/3
  Gain4/1 -> Demux1/1, Add/2
  Demux1/3 -> Mmin/3
  Product1/1 -> Switch1/1  "raw max_ang_acc"
  Demux/4 -> Mmin/4
  1-D Lookup Table1/1 -> Mux2/2  "FR Moment Arm"
  Demux/2 -> Mmin/2
  Mux2/1 -> Aeq/1, Product2/1, Product1/1  "All Moment Arms {FL FR RL RR] (about Vehicle Center of Gravity)"
  Demux/1 -> Mmax/1
  Add/1 -> Demux/1
  Demux1/2 -> Mmax/2
  ub/1 -> Saturation Dynamic2/1, Saturation Dynamic1/1
  Saturation Dynamic1/1 -> Product1/2  "Max TVS Torque"
  Demux1/1 -> Mmin/1
  lb/1 -> Saturation Dynamic2/3, Saturation Dynamic1/3
  Product2/1 -> Switch2/1  "raw min_ang_acc"
  Mmax/1 -> Saturation Dynamic1/2  "Raw Max TVS Torque"
  Constant/1 -> Switch1/3, Gain3/1
  Saturation3/1 -> Sum2/1
  Mmin/1 -> Saturation Dynamic2/2  "Raw Min TVS Torque"
  Saturation Dynamic2/1 -> Product2/2  "Min TVS Torque"
  Divide/1 -> Gain4/1, Add/1  "Equal Torque [FL FR RL RR]"
  Switch1/1 -> Saturation3/1
  Product/1 -> ref_yaw/1, Switch2/2, Switch1/2, Sum1/1  "ref_yaw"
  Constant1/1 -> GreaterThan/2
  steering_angle/1 -> 1-D Lookup Table1/1, Abs1/1, Product3/1, 1-D Lookup Table/1  "Center Column Steering Angle"
  vel/1 -> Selector1/1
  Abs/1 -> 2-D Lookup Table/1
  Product3/1 -> Abs/1, Sign/1
  Sign/1 -> Product/1
  Abs1/1 -> GreaterThan/1
  GreaterThan/1 -> Product3/2
  Selector1/1 -> 2-D Lookup Table/2
  [min_ang_acc] -> Windup Hysteresis/2(min_ang_acc)  "min_ang_acc"
  [max_ang_acc] -> Windup Hysteresis/1(max_ang_acc)  "max_ang_acc"
  [min_ang_acc] -> Saturation Dynamic/3
  [max_ang_acc] -> Saturation Dynamic/1
  Constant5/1 -> Gain5/1
  2-D Lookup Table/1 -> Product/2
  Gain5/1 -> Product/3
  Constant2/1 -> Sum4/1
  Gain2/1 -> Divide/1
  Sum4/1 -> Divide/2

== system car_model_FIXED/Driver & Environment/Longitudinal Control/AAS ==
  v_error : Inport
  Abs : Abs  SaturateOnIntegerOverflow=off
  Constant : Constant
  Discrete-Time Integrator : DiscreteIntegrator  ExternalReset=rising  SampleTime=-1  LimitOutput=on  UpperSaturationLimit=MAX_I_Driver  LowerSaturationLimit=-MAX_I_Driver  ICPrevOutput=DiscIntNeverNeededParam  ICPrevScaledInput=DiscIntNeverNeededParam
  Gain : Gain  Gain=P_Driver
  Gain1 : Gain  Gain=I_Driver
  Less Than : RelationalOperator  Operator=<  OutDataTypeStr=boolean  RndMeth=Simplest  InputSameDT=off
  NOT : Logic  Operator=NOT  IconShape=distinctive  AllPortsSameDT=off  OutDataTypeStr=boolean
  Product : Product
  Saturation : Saturate  UpperLimit=Max_Driver_Input  LowerLimit=Min_Driver_Input
  Sum2 : Sum  Inputs=|++
  driver_input : Outport
  wires:
  Constant/1 -> Less Than/2
  Gain1/1 -> Discrete-Time Integrator/1
  Gain/1 -> Sum2/1
  Sum2/1 -> Saturation/1
  Discrete-Time Integrator/1 -> Sum2/2
  Less Than/1 -> NOT/1, Product/2
  NOT/1 -> Discrete-Time Integrator/2
  Abs/1 -> Less Than/1
  Product/1 -> Gain1/1
  Saturation/1 -> driver_input/1
  v_error/1 -> Abs/1, Product/1, Gain/1  "v_error"
